simulink model "ss1_plant"  (R2019a)
settings: Solver=ode14x  StartTime=0  StopTime=0.456  FixedStep=1e-5  RelTol=1e-3  EnableMultiTasking=on
model workspace (MAT data in the model file):
  Ankle_L_D = 1.86999822456
  Ankle_L_S = 0.0237763920936
  Ankle_R_D = 0.0588397140494
  Ankle_R_S = 0.739584271752
  BeginTimePlantModel = 0.4399
  F_C = 0.06105
  F_H = 0.07
  F_I = 0.00125071180063
  F_L = 0.185
  F_M = 1.13129
  F_W = 0.1
  GRF_HD = 42097.5090581
  GRF_HS = 111995.804745
  GRF_VD = 23523.4518935
  GRF_VS = 88551.3661398
  HAT_I = 3.41998320224
  HAT_L = 0.51264
  HAT_M = 52.89756
  HAT_a = 0.2
  HAT_b = 0.11
  Hip_L_D = 0.00120944164738
  Hip_L_S = 1.91959156409
  Hip_R_D = 0.00174333284727
  Hip_R_S = 0.483982271561
  Knee_L_D = 0.900041230997
  Knee_L_S = 0.0187606009115
  Knee_R_D = 0.0722123401531
  Knee_R_S = 0.0187606009115
  M.stance_ankle = [382.653686523 421.133239746 457.361541748 493.224731445 525.049987793 550.694458008 572.993469238 598.336730957 620.458862305 635.94519043 652.86328125 671.32611084 ... (423 elements, 47x9)]
  M.swing_ankle = [-64.56690979 -57.5369148254 -49.8586082458 -42.14686203 -34.9792785645 -28.8147373199 -23.9411888123 -20.4650421143 -18.3295040131 -17.3495578766 -17.2596321106 -17.7645645142 ... (423 elements, 47x9)]
  M.stance_knee = [185.316421509 185.123703003 166.678710938 142.01902771 126.282310486 108.778045654 87.2157897949 52.3953895569 22.9555110931 -3.17964363098 -32.4531135559 -65.8174972534 ... (423 elements, 47x9)]
  M.swing_knee = [202.892730713 206.914764404 207.933639526 206.428604126 202.740692139 197.00177002 189.179733276 179.200378418 167.046905518 152.816116333 136.765853882 119.338562012 ... (423 elements, 47x9)]
  M.stance_hip = [670.444702148 608.623657227 559.095275879 508.654876709 434.052734375 368.594573975 310.278961182 279.085662842 245.949050903 213.394500732 182.434371948 163.658477783 ... (423 elements, 47x9)]
  M.swing_hip = [-409.603179932 -359.277313232 -304.840881348 -249.20954895 -195.251098633 -145.451843262 -101.693771362 -65.1620788574 -36.3202857971 -14.975810051 -0.45988124609 8.15607261658 ... (423 elements, 47x9)]
  M.stance_ankle_R = [241.344528198; 280.168792725; 315.234191895; 348.458496094; 375.407714844; 399.663421631; 420.77545166; 442.00982666; 462.368896484; 482.825683594; 502.481842041; 523.450317383; 543.702514648; 563.76739502; 584.623718262; 608.33001709; 633.130554199; 657.775634766; 683.749755859; 711.640380859; 738.552185059; 768.736328125; 798.939575195; 830.134277344; 862.95526123; 898.023254395; 934.645629883; 972.008911133; 1011.71954346; 1055.21350098; 1097.53088379; 1139.15075684; 1184.00402832; 1226.12475586; 1272.13769531; 1317.50842285; 1363.38061523; 1410.83459473; 1458.66088867; 1508.37402344; 1555.03942871; 1603.10827637; 1646.82128906; 1687.64489746; 1723.93286133; 1751.32250977; 1770.82592773]
  M.stance_ankle_L = [287.473602295; 320.288269043; 349.08013916; 375.086364746; 395.886169434; 413.086242676; 431.677429199; 447.653686523; 460.621368408; 476.93057251; 488.465698242; 501.313568115; 513.783081055; 527.231506348; 539.797363281; 552.587890625; 569.811767578; 585.799377441; 603.606445312; 624.266845703; 643.495849609; 666.619628906; 688.561279297; 712.704589844; 739.405578613; 766.059448242; 795.171264648; 824.763977051; 856.478515625; 892.682617188; 931.757080078; 975.575866699; 1018.39880371; 1068.90014648; 1121.41381836; 1177.15283203; 1233.20629883; 1294.38818359; 1356.3717041; 1418.45397949; 1482.10351562; 1546.63952637; 1606.78869629; 1662.24047852; 1713.70678711; 1755.8515625; 1788.09362793]
  M.stance_ankle_av = [261.846343994; 297.999664307; 330.276824951; 360.293121338; 384.509216309; 405.629089355; 425.620788574; 444.518188477; 461.592163086; 480.205688477; 496.252441406; 513.611755371; 530.404968262; 547.529174805; 564.700927734; 583.555786133; 604.988952637; 625.786193848; 648.130554199; 672.807739258; 696.304931641; 723.351074219; 749.882568359; 777.94329834; 808.044250488; 839.372680664; 872.657043457; 906.566711426; 942.723388672; 982.977416992; 1023.8536377; 1066.45080566; 1110.4017334; 1156.24707031; 1205.14941406; 1255.12817383; 1305.52526855; 1359.08056641; 1413.19909668; 1468.4095459; 1522.62353516; 1578.0111084; 1629.02905273; 1676.35400391; 1719.38793945; 1753.33544922; 1778.50048828]
  M.swing_ankle_R = [-85.889755249; -81.4323501587; -74.6266021729; -66.0338897705; -56.3612289429; -46.4022369385; -36.9383659363; -28.6265506744; -21.9128284454; -16.9965763092; -13.8461885452; -12.2523727417; -11.90001297; -12.4406614304; -13.5472927094; -14.9475679398; -16.441400528; -17.9046211243; -19.2776374817; -20.5434951782; -21.7070045471; -22.7848415375; -23.8007354736; -24.7754402161; -25.7178401947; -26.6206970215; -27.4531345367; -28.1520080566; -28.6213436127; -28.7432765961; -28.3963775635; -27.4741096497; -25.8983421326; -23.630197525; -20.6837310791; -17.1333255768; -13.1102085114; -8.78991889954; -4.37020587921; -0.0491741187871; 3.98967981339; 7.58726263046; 10.6098003387; 12.9361820221; 14.4380645752; 14.9655628204; 14.3451595306]
  M.swing_ankle_L = [-91.127494812; -88.5172576904; -83.079864502; -75.4265975952; -66.2622070312; -56.3544692993; -46.4767227173; -37.3417816162; -29.5312213898; -23.4348373413; -19.2079906464; -16.7372932434; -15.7042217255; -15.6731481552; -16.1855201721; -16.8559093475; -17.4320354462; -17.8048992157; -17.9840106964; -18.0637702942; -18.1733226776; -18.4301319122; -18.9239711761; -19.703086853; -20.7669734955; -22.0817985535; -23.5756607056; -25.1771774292; -26.8119258881; -28.3871974945; -29.7975158691; -30.9079360962; -31.557094574; -31.5594387054; -30.7291984558; -28.9196014404; -26.046585083; -22.1039409637; -17.1780376434; -11.4525842667; -5.19651222229; 1.25971031189; 7.55906391144; 13.3445072174; 18.2731304169; 22.0209007263; 23.2506732941]
  M.swing_ankle_av = [-88.2176361084; -84.5811920166; -78.3836135864; -70.2084197998; -60.7616653442; -50.8254547119; -41.1776351929; -32.4999885559; -25.2987804413; -19.8580245972; -16.2292098999; -14.2456712723; -13.5907716751; -13.877322197; -14.7198381424; -15.7957201004; -16.8816833496; -17.8603000641; -18.7026901245; -19.4413948059; -20.1364784241; -20.8494167328; -21.6332855225; -22.5210609436; -23.5174541473; -24.6034088135; -25.7298126221; -26.8298587799; -27.8171577454; -28.5850219727; -29.0191078186; -29.0002574921; -28.4133434296; -27.1543045044; -25.1483840942; -22.3716716766; -18.859708786; -14.7072620392; -10.0625753403; -5.11735677719; -0.093072257936; 4.77501726151; 9.25391769409; 13.1176586151; 16.142539978; 18.101266861; 18.3031654358]
  M.stance_knee_R = [304.803405762; 300.279541016; 286.749908447; 260.876068115; 238.10295105; 210.641204834; 181.547897339; 150.171356201; 117.616073608; 82.4058685303; 47.2514076233; 9.42407417297; -24.2061710358; -57.419593811; -89.7506561279; -121.374229431; -150.608276367; -177.107696533; -205.262542725; -233.704879761; -258.570648193; -287.401275635; -315.001159668; -341.735992432; -368.986816406; -397.352233887; -429.581481934; -461.832946777; -494.10635376; -527.185058594; -559.887207031; -588.972290039; -619.081665039; -645.119018555; -673.582641602; -697.401916504; -718.140319824; -735.778747559; -747.575012207; -758.092407227; -758.573730469; -756.998291016; -746.309448242; -733.501403809; -711.673217773; -684.145324707; -652.518432617]
  M.stance_knee_L = [243.44644165; 255.942733765; 248.447509766; 236.900390625; 224.860092163; 212.20489502; 192.68132019; 170.520477295; 148.683563232; 121.948730469; 95.7874603271; 68.55103302; 42.090297699; 13.6919345856; -12.3652801514; -38.7850036621; -64.9619522095; -88.0590744019; -112.283294678; -133.897094727; -155.896942139; -177.537506104; -199.712860107; -222.443725586; -246.961090088; -269.91027832; -297.39855957; -322.404815674; -347.004272461; -374.282318115; -397.260803223; -423.561889648; -443.694885254; -465.390808105; -484.542419434; -506.723937988; -523.60723877; -539.251403809; -553.182617188; -561.621337891; -567.393188477; -571.484802246; -571.686096191; -565.345947266; -556.19708252; -540.071105957; -519.244873047]
  M.stance_knee_av = [277.533630371; 280.574310303; 269.726623535; 250.220214844; 232.217224121; 211.336181641; 186.49609375; 159.215408325; 131.423858643; 99.98046875; 68.8229904175; 35.7027206421; 5.25892496109; -25.8144702911; -55.3571586609; -84.6679153442; -112.543243408; -137.530532837; -163.938446045; -189.345840454; -212.937911987; -238.572921753; -263.761932373; -288.717193604; -314.753173828; -340.711364746; -370.833557129; -399.864898682; -428.727661133; -459.228302002; -487.608825684; -515.456542969; -541.131958008; -565.239746094; -589.564758301; -612.656066895; -631.681152344; -648.433227539; -661.178405762; -670.771911621; -673.604614258; -674.547729492; -668.699035645; -658.765625; -642.572753906; -620.112365723; -593.285766602]
  M.swing_knee_R = [199.516082764; 210.401519775; 215.828033447; 216.27961731; 212.701660156; 206.257568359; 198.006378174; 188.676239014; 178.593338013; 167.751281738; 155.966705322; 143.082733154; 129.140670776; 114.425209045; 99.4022216797; 84.6166915894; 70.5888824463; 57.7218399048; 46.2420120239; 36.183429718; 27.4012203217; 19.5964603424; 12.3447122574; 5.1349864006; -2.6006064415; -11.4854259491; -22.1804237366; -35.3444290161; -51.6237678528; -71.6230010986; -95.8606109619; -124.642044067; -157.887771606; -194.970367432; -234.706756592; -275.472839355; -315.379730225; -352.45715332; -384.76776123; -410.475341797; -427.916656494; -435.71270752; -432.9347229; -419.276306152; -395.139343262; -361.678741455; -320.789794922]
  M.swing_knee_L = [164.096496582; 181.32963562; 193.40145874; 200.345535278; 202.785949707; 201.703689575; 198.146636963; 192.944168091; 186.504760742; 178.839569092; 169.754180908; 159.021072388; 146.566345215; 132.544692993; 117.362823486; 101.647209167; 86.1308898926; 71.517906189; 58.3772506714; 47.1123123169; 37.946975708; 30.9007816315; 25.7909584045; 22.2543544769; 19.7833538055; 17.7391624451; 15.3230056763; 11.6997699738; 6.09846830368; -2.1977686882; -13.9393539429; -29.9818992615; -51.2079772949; -78.3828964233; -111.999908447; -152.125411987; -198.241424561; -249.101135254; -302.666015625; -356.14050293; -406.130554199; -448.915588379; -480.807739258; -498.666107178; -500.297241211; -484.827392578; -454.950439453]
  M.swing_knee_av = [367.548095703; 394.961334229; 411.721313477; 418.395629883; 416.589355469; 408.467224121; 396.137420654; 381.146179199; 364.219024658; 345.358825684; 324.188934326; 300.332885742; 273.770843506; 244.956619263; 214.769424438; 184.371643066; 154.992874146; 127.706855774; 103.270904541; 82.0814208984; 64.1764450073; 49.2412033081; 36.6416435242; 25.4871902466; 14.6956396103; 3.0065600872; -5.51223230362; -14.4358959198; -25.9694404602; -40.7673416138; -59.4511642456; -82.5708694458; -110.474525452; -143.1537323; -180.170394897; -220.651763916; -263.318267822; -306.521148682; -348.278106689; -386.326507568; -418.233947754; -441.580657959; -454.211608887; -454.560668945; -441.876159668; -416.411499023; -380.416778564]
  M.stance_hip_R = [677.309082031; 662.534851074; 638.490905762; 616.795959473; 568.749938965; 517.141235352; 455.908843994; 395.977142334; 341.056732178; 296.010314941; 256.942687988; 232.045257568; 207.015548706; 187.887771606; 172.106338501; 157.565826416; 140.384109497; 121.182800293; 105.588790894; 91.3845062256; 72.1999969482; 60.2186164856; 45.7028198242; 30.413274765; 15.0268573761; 0.406857311726; -7.57483196259; -15.6972227097; -25.5365505219; -37.0106239319; -47.2925415039; -63.028678894; -78.3000335693; -97.126083374; -112.66633606; -133.688415527; -158.219207764; -186.10067749; -222.072463989; -257.30267334; -303.991699219; -349.784912109; -402.389801025; -448.147857666; -499.237121582; -543.315307617; -578.758666992]
  M.stance_hip_L = [543.206542969; 533.482299805; 548.817321777; 551.911437988; 531.989379883; 493.179870605; 449.218536377; 400.603149414; 345.233306885; 294.070343018; 246.907104492; 206.114685059; 169.324005127; 144.570343018; 122.85004425; 107.517539978; 94.4359436035; 78.0879211426; 64.8094940186; 47.6538200378; 33.5419006348; 17.3963489532; 5.34900474548; -6.64071655273; -16.2073192596; -27.9363861084; -31.1544418335; -38.8874778748; -46.7718048096; -50.9772720337; -62.9813499451; -70.4582366943; -86.7793121338; -104.007881165; -125.457344055; -142.477386475; -168.722595215; -199.240997314; -232.18812561; -274.7059021; -320.62008667; -367.697479248; -414.968200684; -465.465026855; -512.790344238; -558.792602539; -597.835327148]
  M.stance_hip_av = [617.707946777; 605.178161621; 598.635986328; 587.958374023; 552.411865234; 506.491699219; 452.935394287; 398.03314209; 342.912994385; 295.148101807; 252.482421875; 220.520568848; 190.263763428; 168.635574341; 150.214660645; 135.322143555; 119.96269989; 102.029510498; 87.4646606445; 71.9486465454; 55.0186271667; 41.1864967346; 27.767791748; 13.9448347092; 1.1450009346; -12.1901378632; -18.0546607971; -26.0040035248; -34.9744415283; -43.2180213928; -54.2653427124; -66.3307037354; -82.0686035156; -100.184661865; -118.351226807; -137.59463501; -162.887359619; -191.940826416; -226.568313599; -265.037445068; -311.382110596; -357.746063232; -407.980194092; -455.844390869; -505.260803223; -550.194091797; -587.237182617]
  M.swing_hip_R = [-538.103820801; -497.101409912; -442.370605469; -376.893707275; -304.863922119; -231.227020264; -160.946350098; -98.2951431274; -46.3001785278; -6.44236755371; 21.340795517; 38.314250946; 46.3760261536; 47.5502052307; 43.6576118469; 36.0970802307; 25.7352046967; 12.9887065887; -1.99190557003; -19.1645908356; -38.4166030884; -59.3577880859; -81.1436386108; -102.423095703; -121.337936401; -135.433135986; -141.69631958; -136.773361206; -117.19405365; -79.869178772; -22.6713924408; 54.7419433594; 150.165710449; 258.460906982; 372.17489624; 482.859954834; 582.569580078; 665.075012207; 726.33203125; 764.304260254; 778.477111816; 769.368469238; 738.280151367; 687.311401367; 619.35723877; 538.24987793; 448.937438965]
  M.swing_hip_L = [-461.667541504; -443.129730225; -412.952697754; -372.32824707; -323.551696777; -269.754852295; -214.532669067; -161.444091797; -113.441833496; -72.5716552734; -39.8347740173; -15.1222686768; 2.44718074799; 14.1845970154; 21.4651794434; 25.459356308; 27.0601558685; 26.8279724121; 24.9684696198; 21.2653636932; 15.2047595978; 6.27575731277; -5.8063416481; -20.9604568481; -38.6427841187; -57.7537269592; -76.4598388672; -92.4824371338; -103.319824219; -106.302307129; -98.579864502; -77.1716766357; -39.4084091187; 16.4871692657; 90.8427581787; 182.152694702; 286.93371582; 399.804718018; 513.893920898; 621.449401855; 714.596923828; 786.088867188; 829.926391602; 842.146728516; 821.168579102; 768.122131348; 691.412231445]
  M.swing_hip_av = [-504.132110596; -473.113983154; -429.29598999; -374.864593506; -313.169586182; -248.350509644; -184.762496948; -126.361343384; -76.1409072876; -35.8331642151; -5.84834623337; 14.5646886826; 26.8520946503; 32.7210464478; 33.7943077087; 31.3692054749; 26.3240718842; 19.1394901276; 9.99048233032; -1.19572210312; -14.5848884583; -30.1873207092; -47.6603965759; -66.2174758911; -84.5845413208; -100.908950806; -112.702316284; -117.088516235; -111.027740479; -91.6172332764; -56.4084892273; -3.88633561134; 65.9105529785; 150.917037964; 247.138397217; 349.212280273; 451.17590332; 547.177124023; 631.915161133; 700.813171387; 750.08581543; 776.799743652; 779.01184082; 756.12713623; 709.051147461; 640.415344238; 556.704040527]
  S_I = 0.0556212184297
  S_L = 0.41
  S_M = 3.62793
  S_R1 = 0.035
  S_R2 = 0.0716197243914
  T_I = 0.63371745
  T_L = 0.6
  T_M = 7.802
  T_R1 = 0.0716197243914
  T_R2 = 0.105042262441
  bodymass = 78.02
  p_stance_ankle = 3.52408223904
  p_stance_hip = 23.8147315857
  p_stance_knee = -14.6270017634
  p_swing_ankle = -34.807471817
  p_swing_hip = -19.0751814577
  p_swing_knee = -0.719736499265
  polyfit_stance_ankle = [7.25005766341 -2.94260084728 3.61751641686 -0.1600680665]
  polyfit_swing_ankle = [-11368.0037517 20285.4827832 -14825.218273 5697.61347658 -1221.0674564 140.988649334 -7.60353693637 0.110238664523]
  polyfit_swing_hip = [-6497.04836191 6353.1189755 -1512.41069047 -218.046365216 114.745718447 -9.14187395017 -0.14056630138]
  polyfit_swing_knee = [20801.7792641 -51031.8985583 53804.8965773 -29864.6420618 9069.83319333 -1458.09150169 107.955966741 -2.65469998779 0.0787369748099]
  stance_hip_D = -0.2
  stance_hip_I = 0
  stance_hip_P = -2
  stance_knee_D = 0.1
  stance_knee_I = 0
  stance_knee_P = 1
  u_stance_ankle = [2.09207920849e-06 2.83402277191e-05 -1.09458664945e-06 -2.15225634711e-07 1.00199670569e-07 -0.0321391439721]
  u_swing_ankle = [-0.000249118459232 -0.000670477458577 -0.000829633071132 -0.000874405796854 -0.000839016598733 -0.000796307977786]
  u_swing_hip = [-0.00160905629459 -0.00453587585235 -0.00786706006827 -0.000770525358696 -0.0150520831351 -0.0149081405775]
  u_swing_knee = [6.43563712018e-07 -4.04341590665e-07 7.15097641992e-07 -6.45757706781e-07 -0.0441867306802 -2.32579449741e-08]
  w_stance_ankle = 15.4408631407
  w_stance_hip = -43.933457531
  w_stance_knee = -25.2069201526
  w_swing_ankle = -15.2
  w_swing_hip = 136.9
  w_swing_knee = -386.2
undefined symbols (not defined in the file or in its folder): X, Y, Z
libraries: nesl_utility x81, sm_lib x49, fl_lib x24, fl_ps_legacy_lib x16
(part 1 of 7)
settings Model: OrderedModelArguments=off  Creator=6438sunj  LastModifiedBy=jess-local
settings DataIOCC: LimitDataPoints=on  SaveFormat=Array  SignalLoggingSaveFormat=ModelDataLogs  ReturnWorkspaceOutputs=off  SignalLoggingName=SPE_DataLog  OutputOption=SpecifiedOutputTimes  OutputTimes=spe_config.time
settings OptimizationCC: ExpressionDepthLimit=2147483647  LifeSpan=inf
settings DebuggingCC: UnderspecifiedInitializationDetection=Classic  MergeDetectMultiDrivingBlocksExec=none  SolverPrmCheckMsg=warning  StateNameClashWarn=warning  SFUnexpectedBacktrackingDiag=warning  SFNoUnconditionalDefaultTransitionDiag=warning  SFExecutionAtInitializationDiag=none  ArithmeticOperatorsInVariantConditions=warning
settings HardwareCC: ProdBitPerPointer=32  ProdBitPerSizeT=32  ProdBitPerPtrDiffT=32  ProdLargestAtomicFloat=None  ProdIntDivRoundTo=Undefined  ProdEndianess=Unspecified  ProdWordSize=32  ProdHWDeviceType=32-bit Generic
settings ModelReferenceCC: PropagateSignalLabelsOutOfModel=off
settings SFSimCC: SimUseLocalCustomCode=off
settings RTWCC: RTWUseLocalCustomCode=off
settings CodeAppCC: StateflowObjectComments=on
settings GRTTargetCC: TargetLangStandard=C89/C90 (ANSI)  GeneratePreprocessorConditionals=Disable all
settings ConfigComp: CovMetricSettings=dw  CovHtmlReporting=on  CovSaveCumulativeToWorkspaceVar=on  CovSaveSingleToWorkspaceVar=on  CovExternalEMLEnable=off
settings SimscapeCC: SimscapeNormalizeSystem=off
settings ConfigurationSet: Description=SimMechanics 2G
settings DiagnosticsConfigSet: SimMechanicsUnconnectedFramePorts=none
settings ExplorerConfigSet: InternalSimMechanicsExplorerSettings="<ExplorerConfiguration><canonicalview>default</canonicalview><TilePanel><TileInfo><Tiles Columns=\"1\" Count=\"1\" Rows=\"1\"><Column Left=\"2\" Weight=\"1\"/><Column Left=\"715\"/><Row Top=\"2\" Weight=\"1\"/><Row Top=\"555\"/><Tile Height=\"1\" Width=\"1\" X=\"0\" Y=\"0\"/></Tiles></TileInfo><SceneInfo><SceneViewer><BGColor><R>0.60000002384185791</R><G>0.60000002384185791</G><B>0.60000002384185791</B></BGColor><Camera><Position><X>2.3238188926266905</X><Y>0.29801581507321606</Y><Z>0.5830879823253462</Z></Position><Center><X>0</X><Y>0.29801581507321606</Y><Z>0.5830879823253462</Z></Center><Up><X>-0</X><Y>0</Y><Z>1</Z></Up><Left>-0.37797235250473021</Left><Right>0.37797235250473021</Right><Bottom>-0.82692947387695315</Bottom><Top>0.82692947387695315</Top></Camera></SceneViewer></SceneInfo></TilePanel></ExplorerConfiguration>"

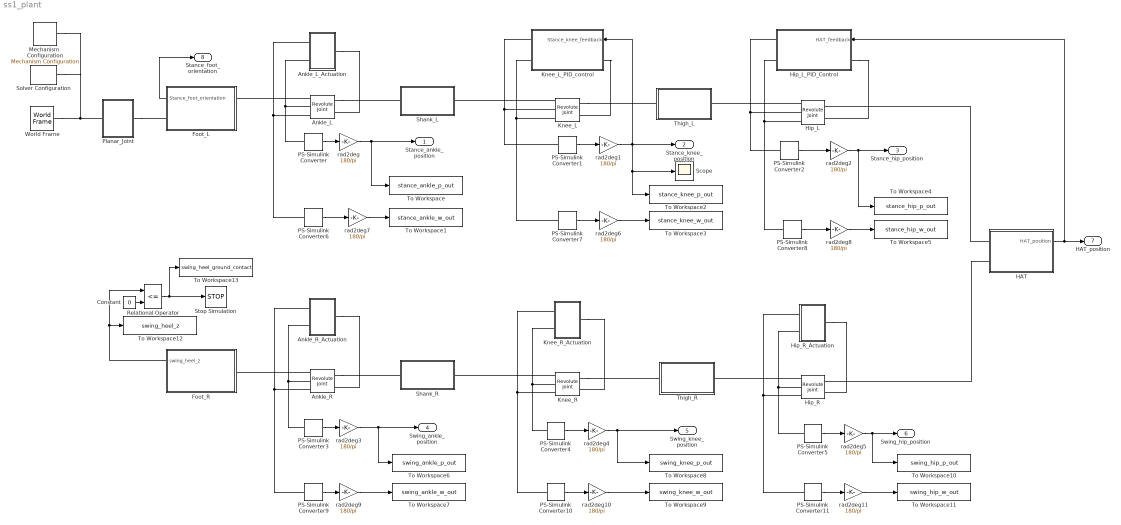
== system ss1_plant ==
  Ankle_L : sm_lib/Joints/Revolute Joint  SenseConstraintForce=off  SenseConstraintForceX=off  SenseConstraintForceY=off  SenseConstraintForceZ=off  SenseConstraintTorque=off  SenseConstraintTorqueX=off  SenseConstraintTorqueY=off  SenseConstraintTorqueZ=off  SenseTotalForce=off  SenseTotalForceX=off  SenseTotalForceY=off  SenseTotalForceZ=off  SenseTotalTorque=off  SenseTotalTorqueX=off  SenseTotalTorqueY=off  SenseTotalTorqueZ=off  CompositeWrenchDir=FollowerOnBase  CompositeWrenchFrame=BaseFrame  EquilibriumPosition=0  EquilibriumPositionUnits=deg  SpringStiffness=Ankle_L_S  SpringStiffnessUnits=N*m/deg  DampingCoefficient=Ankle_L_D  DampingCoefficientUnits=N*m/(deg/s)  TorqueActuationMode=InputTorque  MotionActuationMode=ComputedMotion  SensePosition=on  SenseVelocity=on  SenseAcceleration=off  SenseTorqueForce=off  SenseLowerLimitTorqueForce=off  SenseUpperLimitTorqueForce=off  LowerLimitSpecify=off  LowerLimitBound=-90  LowerLimitBoundUnits=deg  LowerLimitStiffness=1e4  LowerLimitStiffnessUnits=N*m/deg  LowerLimitDamping=10  LowerLimitDampingUnits=N*m/(deg/s)  LowerLimitTransitionRegionWidth=0.1  LowerLimitTransitionRegionWidthUnits=deg  UpperLimitSpecify=off  UpperLimitBound=90  UpperLimitBoundUnits=deg  UpperLimitStiffness=1e4  UpperLimitStiffnessUnits=N*m/deg  UpperLimitDamping=10  UpperLimitDampingUnits=N*m/(deg/s)  UpperLimitTransitionRegionWidth=0.1  UpperLimitTransitionRegionWidthUnits=deg  PositionTargetSpecify=on  PositionTargetPriority=High  PositionTargetValue=p_stance_ankle  PositionTargetValueUnits=deg  VelocityTargetSpecify=on  VelocityTargetPriority=High  VelocityTargetValue=w_stance_ankle  VelocityTargetValueUnits=deg/s
  Ankle_L_Actuation : Subsystem
  Ankle_R : sm_lib/Joints/Revolute Joint  SenseConstraintForce=off  SenseConstraintForceX=off  SenseConstraintForceY=off  SenseConstraintForceZ=off  SenseConstraintTorque=off  SenseConstraintTorqueX=off  SenseConstraintTorqueY=off  SenseConstraintTorqueZ=off  SenseTotalForce=off  SenseTotalForceX=off  SenseTotalForceY=off  SenseTotalForceZ=off  SenseTotalTorque=off  SenseTotalTorqueX=off  SenseTotalTorqueY=off  SenseTotalTorqueZ=off  CompositeWrenchDir=FollowerOnBase  CompositeWrenchFrame=BaseFrame  EquilibriumPosition=0  EquilibriumPositionUnits=deg  SpringStiffness=Ankle_R_S  SpringStiffnessUnits=N*m/deg  DampingCoefficient=Ankle_R_D  DampingCoefficientUnits=N*m/(deg/s)  TorqueActuationMode=InputTorque  MotionActuationMode=ComputedMotion  SensePosition=on  SenseVelocity=on  SenseAcceleration=off  SenseTorqueForce=off  SenseLowerLimitTorqueForce=off  SenseUpperLimitTorqueForce=off  LowerLimitSpecify=off  LowerLimitBound=-90  LowerLimitBoundUnits=deg  LowerLimitStiffness=1e4  LowerLimitStiffnessUnits=N*m/deg  LowerLimitDamping=10  LowerLimitDampingUnits=N*m/(deg/s)  LowerLimitTransitionRegionWidth=0.1  LowerLimitTransitionRegionWidthUnits=deg  UpperLimitSpecify=off  UpperLimitBound=90  UpperLimitBoundUnits=deg  UpperLimitStiffness=1e4  UpperLimitStiffnessUnits=N*m/deg  UpperLimitDamping=10  UpperLimitDampingUnits=N*m/(deg/s)  UpperLimitTransitionRegionWidth=0.1  UpperLimitTransitionRegionWidthUnits=deg  PositionTargetSpecify=on  PositionTargetPriority=High  PositionTargetValue=p_swing_ankle  PositionTargetValueUnits=deg  VelocityTargetSpecify=on  VelocityTargetPriority=High  VelocityTargetValue=w_swing_ankle  VelocityTargetValueUnits=deg/s
  Ankle_R_Actuation : Subsystem
  Constant : Constant  Value=0
  Foot_L : Subsystem  mask{F_L=F_L, F_H=F_H, F_C=F_C, F_W=F_W, F_M=F_M, F_I=F_I}
      mask prompts: F_L "Foot Length (m)"; F_H "Foot Height (m)"; F_C "Heel to Mid Foot (m)"; F_W "Foot Width (m)"; F_M "Foot Mass (kg)"; F_I "Foot Moment of Inertia (kg*m^2)"
      mask init:
      | % Defines the cross section of the thigh
      | 
      | F_cross_section = [(F_L-F_C),0;0, F_H; -F_C,0 ];
  Foot_R : Subsystem  mask{F_L=F_L, F_H=F_H, F_C=F_C, F_W=F_W, F_M=F_M, F_I=F_I}
      mask prompts: F_L "Foot Length (m)"; F_H "Foot Height (m)"; F_C "Heel to Mid Foot (m)"; F_W "Foot Width (m)"; F_M "Foot Mass (kg)"; F_I "Foot Moment of Inertia (kg*m^2)"
      mask init:
      | % Defines the cross section of the thigh
      | 
      | F_cross_section = [(F_L-F_C),0;0, F_H; -F_C,0; ];
  HAT : Subsystem  mask{HAT_a=HAT_a, HAT_b=HAT_b, HAT_L=HAT_L, HAT_M=HAT_M, HAT_I=HAT_I}
      mask prompts: HAT_a "Long Axis Length (m)"; HAT_b "Short Axis Length (m)"; HAT_L "HAT Height (m)"; HAT_M "Mass (kg)"; HAT_I "Moment of Inertia (kg*m^2)"
      mask init:
      | % Defines the cross-section of the HAT
      | theta = ([0:.01:360]*(pi/180))';
      | HAT_cross_section = [HAT_a*cos(theta), HAT_b*sin(theta)];
  Hip_L : sm_lib/Joints/Revolute Joint  SenseConstraintForce=off  SenseConstraintForceX=off  SenseConstraintForceY=off  SenseConstraintForceZ=off  SenseConstraintTorque=off  SenseConstraintTorqueX=off  SenseConstraintTorqueY=off  SenseConstraintTorqueZ=off  SenseTotalForce=off  SenseTotalForceX=off  SenseTotalForceY=off  SenseTotalForceZ=off  SenseTotalTorque=off  SenseTotalTorqueX=off  SenseTotalTorqueY=off  SenseTotalTorqueZ=off  CompositeWrenchDir=FollowerOnBase  CompositeWrenchFrame=BaseFrame  EquilibriumPosition=0  EquilibriumPositionUnits=deg  SpringStiffness=Hip_L_S  SpringStiffnessUnits=N*m/deg  DampingCoefficient=Hip_L_D  DampingCoefficientUnits=N*m/(deg/s)  TorqueActuationMode=InputTorque  MotionActuationMode=ComputedMotion  SensePosition=on  SenseVelocity=on  SenseAcceleration=off  SenseTorqueForce=off  SenseLowerLimitTorqueForce=off  SenseUpperLimitTorqueForce=off  LowerLimitSpecify=off  LowerLimitBound=-90  LowerLimitBoundUnits=deg  LowerLimitStiffness=1e4  LowerLimitStiffnessUnits=N*m/deg  LowerLimitDamping=10  LowerLimitDampingUnits=N*m/(deg/s)  LowerLimitTransitionRegionWidth=0.1  LowerLimitTransitionRegionWidthUnits=deg  UpperLimitSpecify=off  UpperLimitBound=90  UpperLimitBoundUnits=deg  UpperLimitStiffness=1e4  UpperLimitStiffnessUnits=N*m/deg  UpperLimitDamping=10  UpperLimitDampingUnits=N*m/(deg/s)  UpperLimitTransitionRegionWidth=0.1  UpperLimitTransitionRegionWidthUnits=deg  PositionTargetSpecify=on  PositionTargetPriority=High  PositionTargetValue=p_stance_hip  PositionTargetValueUnits=deg  VelocityTargetSpecify=on  VelocityTargetPriority=High  VelocityTargetValue=w_stance_hip  VelocityTargetValueUnits=deg/s
  Hip_L_PID_Control : Subsystem
  Hip_R : sm_lib/Joints/Revolute Joint  SenseConstraintForce=off  SenseConstraintForceX=off  SenseConstraintForceY=off  SenseConstraintForceZ=off  SenseConstraintTorque=off  SenseConstraintTorqueX=off  SenseConstraintTorqueY=off  SenseConstraintTorqueZ=off  SenseTotalForce=off  SenseTotalForceX=off  SenseTotalForceY=off  SenseTotalForceZ=off  SenseTotalTorque=off  SenseTotalTorqueX=off  SenseTotalTorqueY=off  SenseTotalTorqueZ=off  CompositeWrenchDir=FollowerOnBase  CompositeWrenchFrame=BaseFrame  EquilibriumPosition=0  EquilibriumPositionUnits=deg  SpringStiffness=Hip_R_S  SpringStiffnessUnits=N*m/deg  DampingCoefficient=Hip_R_D  DampingCoefficientUnits=N*m/(deg/s)  TorqueActuationMode=InputTorque  MotionActuationMode=ComputedMotion  SensePosition=on  SenseVelocity=on  SenseAcceleration=off  SenseTorqueForce=off  SenseLowerLimitTorqueForce=off  SenseUpperLimitTorqueForce=off  LowerLimitSpecify=off  LowerLimitBound=-90  LowerLimitBoundUnits=deg  LowerLimitStiffness=1e4  LowerLimitStiffnessUnits=N*m/deg  LowerLimitDamping=10  LowerLimitDampingUnits=N*m/(deg/s)  LowerLimitTransitionRegionWidth=0.1  LowerLimitTransitionRegionWidthUnits=deg  UpperLimitSpecify=off  UpperLimitBound=90  UpperLimitBoundUnits=deg  UpperLimitStiffness=1e4  UpperLimitStiffnessUnits=N*m/deg  UpperLimitDamping=10  UpperLimitDampingUnits=N*m/(deg/s)  UpperLimitTransitionRegionWidth=0.1  UpperLimitTransitionRegionWidthUnits=deg  PositionTargetSpecify=on  PositionTargetPriority=High  PositionTargetValue=p_swing_hip  PositionTargetValueUnits=deg  VelocityTargetSpecify=on  VelocityTargetPriority=High  VelocityTargetValue=w_swing_hip  VelocityTargetValueUnits=deg/s
  Hip_R_Actuation : Subsystem
  Knee_L : sm_lib/Joints/Revolute Joint  SenseConstraintForce=off  SenseConstraintForceX=off  SenseConstraintForceY=off  SenseConstraintForceZ=off  SenseConstraintTorque=off  SenseConstraintTorqueX=off  SenseConstraintTorqueY=off  SenseConstraintTorqueZ=off  SenseTotalForce=off  SenseTotalForceX=off  SenseTotalForceY=off  SenseTotalForceZ=off  SenseTotalTorque=off  SenseTotalTorqueX=off  SenseTotalTorqueY=off  SenseTotalTorqueZ=off  CompositeWrenchDir=FollowerOnBase  CompositeWrenchFrame=BaseFrame  EquilibriumPosition=0  EquilibriumPositionUnits=deg  SpringStiffness=Knee_L_S  SpringStiffnessUnits=N*m/deg  DampingCoefficient=Knee_L_D  DampingCoefficientUnits=N*m/(deg/s)  TorqueActuationMode=InputTorque  MotionActuationMode=ComputedMotion  SensePosition=on  SenseVelocity=on  SenseAcceleration=off  SenseTorqueForce=off  SenseLowerLimitTorqueForce=off  SenseUpperLimitTorqueForce=off  LowerLimitSpecify=off  LowerLimitBound=-90  LowerLimitBoundUnits=deg  LowerLimitStiffness=1e4  LowerLimitStiffnessUnits=N*m/deg  LowerLimitDamping=10  LowerLimitDampingUnits=N*m/(deg/s)  LowerLimitTransitionRegionWidth=0.1  LowerLimitTransitionRegionWidthUnits=deg  UpperLimitSpecify=off  UpperLimitBound=90  UpperLimitBoundUnits=deg  UpperLimitStiffness=1e4  UpperLimitStiffnessUnits=N*m/deg  UpperLimitDamping=10  UpperLimitDampingUnits=N*m/(deg/s)  UpperLimitTransitionRegionWidth=0.1  UpperLimitTransitionRegionWidthUnits=deg  PositionTargetSpecify=on  PositionTargetPriority=High  PositionTargetValue=p_stance_knee  PositionTargetValueUnits=deg  VelocityTargetSpecify=on  VelocityTargetPriority=High  VelocityTargetValue=w_stance_knee  VelocityTargetValueUnits=deg/s
  Knee_L_PID_control : Subsystem
  Knee_R : sm_lib/Joints/Revolute Joint  SenseConstraintForce=off  SenseConstraintForceX=off  SenseConstraintForceY=off  SenseConstraintForceZ=off  SenseConstraintTorque=off  SenseConstraintTorqueX=off  SenseConstraintTorqueY=off  SenseConstraintTorqueZ=off  SenseTotalForce=off  SenseTotalForceX=off  SenseTotalForceY=off  SenseTotalForceZ=off  SenseTotalTorque=off  SenseTotalTorqueX=off  SenseTotalTorqueY=off  SenseTotalTorqueZ=off  CompositeWrenchDir=FollowerOnBase  CompositeWrenchFrame=BaseFrame  EquilibriumPosition=0  EquilibriumPositionUnits=deg  SpringStiffness=Knee_R_S  SpringStiffnessUnits=N*m/deg  DampingCoefficient=Knee_R_D  DampingCoefficientUnits=N*m/(deg/s)  TorqueActuationMode=InputTorque  MotionActuationMode=ComputedMotion  SensePosition=on  SenseVelocity=on  SenseAcceleration=off  SenseTorqueForce=off  SenseLowerLimitTorqueForce=off  SenseUpperLimitTorqueForce=off  LowerLimitSpecify=off  LowerLimitBound=-90  LowerLimitBoundUnits=deg  LowerLimitStiffness=1e4  LowerLimitStiffnessUnits=N*m/deg  LowerLimitDamping=10  LowerLimitDampingUnits=N*m/(deg/s)  LowerLimitTransitionRegionWidth=0.1  LowerLimitTransitionRegionWidthUnits=deg  UpperLimitSpecify=off  UpperLimitBound=90  UpperLimitBoundUnits=deg  UpperLimitStiffness=1e4  UpperLimitStiffnessUnits=N*m/deg  UpperLimitDamping=10  UpperLimitDampingUnits=N*m/(deg/s)  UpperLimitTransitionRegionWidth=0.1  UpperLimitTransitionRegionWidthUnits=deg  PositionTargetSpecify=on  PositionTargetPriority=High  PositionTargetValue=p_swing_knee  PositionTargetValueUnits=deg  VelocityTargetSpecify=on  VelocityTargetPriority=High  VelocityTargetValue=w_swing_knee  VelocityTargetValueUnits=deg/s
  Knee_R_Actuation : Subsystem
  Mechanism  Configuration : sm_lib/Utilities/Mechanism Configuration  UniformGravity=Constant  GravityVector=[0 0 -9.81]  GravityUnits=m/s^2  LinearizationDelta=0.001
  PS-Simulink Converter{,1..11} (12 alike) : nesl_utility/PS-Simulink Converter  PhysicalDomain=network_engine_domain  SubClassName=ps_output  LeftPortType=input  RightPortType=output  PseudoPeriodic=off  Frequencies=[]  Unit=1  AffineConversion=off
  Planar_Joint : Subsystem
  Relational Operator : RelationalOperator  Operator=<=  OutDataTypeStr=boolean  RndMeth=Simplest
  Scope : Scope
  Shank_L : Subsystem  mask{S_R2=S_R2, S_R1=S_R1, S_L=S_L, S_M=S_M, S_I=S_I}
      mask prompts: S_R2 "Proximal End Radius (m)"; S_R1 "Distal End Radius (m)"; S_L "Shank Length (m)"; S_M "Shank Mass (kg)"; S_I "Shank Moment of Inertia (kg*m^2)"
      mask init:
      | % Defines the cross section of the thigh
      | 
      | S_cross_section = [0,0; S_R1, 0; S_R2, S_L; 0,S_L];
  Shank_R : Subsystem  mask{S_R2=S_R2, S_R1=S_R1, S_L=S_L, S_M=S_M, S_I=S_I}
      mask prompts: S_R2 "Proximal End Radius (m)"; S_R1 "Distal End Radius (m)"; S_L "Shank Length (m)"; S_M "Shank Mass (kg)"; S_I "Shank Moment of Inertia (kg*m^2)"
      mask init:
      | % Defines the cross section of the thigh
      | 
      | S_cross_section = [0,0; S_R1, 0; S_R2, S_L; 0,S_L];
  Solver Configuration : nesl_utility/Solver Configuration  PhysicalDomain=network_engine_domain  SubClassName=solver  LeftPortType=input  RightPortType=generic  Tones=[]  Harmonics=[]  SimulateNoise=off  Profile=off  UseLocalSampling=off  EnableSwitchedLinearOptims=on  FrequencyDomain=off  UseCCode=off  RelTol=0.001  AbsTol=1e-06  MinStep=1e-09  ToWorkspace=off  RevertToSquareIcSolve=off  NumHomotopyIterations=100  PhasorMode=off  PhasorModeNumHarmonics=1  DoDC=off  ResidualTolerance=1e-9  UseLocalSolver=off  LocalSolverChoice=NE_BACKWARD_EULER_ADVANCER  LocalSolverSampleTime=.001  DoFixedCost=off  MaxNonlinIter=3  MaxModeIter=2  LinearAlgebra=Sparse  EquationFormulation=NE_TIME_EF  DelaysMemoryBudget=1024  AutomaticFiltering=on  FilteringTimeConstant=0.001  PartitionStorageMethod=AS_NEEDED  PartitionMemoryBudget=1024  PartitionMethod=FAST
  Stop Simulation : Stop
  Thigh_L : Subsystem  mask{T_R2=T_R2, T_R1=T_R1, T_L=T_L, T_M=T_M, T_I=T_I}
      mask prompts: T_R2 "Proximal End Radius (m)"; T_R1 "Distal End Radius (m)"; T_L "Thigh Length (m)"; T_M "Thigh Mass (kg)"; T_I "Thigh Moment of Inertia (kg*m^2)"
      mask init:
      | % Defines the cross section of the thigh
      | 
      | T_cross_section = [0,0; T_R1, 0; T_R2, T_L; 0,T_L];
  Thigh_R : Subsystem  mask{T_R2=T_R2, T_R1=T_R1, T_L=T_L, T_M=T_M, T_I=T_I}
      mask prompts: T_R2 "Proximal End Radius (m)"; T_R1 "Distal End Radius (m)"; T_L "Thigh Length (m)"; T_M "Thigh Mass (kg)"; T_I "Thigh Moment of Inertia (kg*m^2)"
      mask init:
      | % Defines the cross section of the thigh
      | 
      | T_cross_section = [0,0; T_R1, 0; T_R2, T_L; 0,T_L];
  To Workspace : ToWorkspace  VariableName=stance_ankle_p_out  SampleTime=-1
  To Workspace1 : ToWorkspace  VariableName=stance_ankle_w_out  SampleTime=-1
  To Workspace10 : ToWorkspace  VariableName=swing_hip_p_out  SampleTime=-1
  To Workspace11 : ToWorkspace  VariableName=swing_hip_w_out  SampleTime=-1
  To Workspace12 : ToWorkspace  VariableName=swing_heel_z  SampleTime=-1
  To Workspace13 : ToWorkspace  VariableName=swing_heel_ground_contact  SampleTime=-1
  To Workspace2 : ToWorkspace  VariableName=stance_knee_p_out  SampleTime=-1
  To Workspace3 : ToWorkspace  VariableName=stance_knee_w_out  SampleTime=-1
  To Workspace4 : ToWorkspace  VariableName=stance_hip_p_out  SampleTime=-1
  To Workspace5 : ToWorkspace  VariableName=stance_hip_w_out  SampleTime=-1
  To Workspace6 : ToWorkspace  VariableName=swing_ankle_p_out  SampleTime=-1
  To Workspace7 : ToWorkspace  VariableName=swing_ankle_w_out  SampleTime=-1
  To Workspace8 : ToWorkspace  VariableName=swing_knee_p_out  SampleTime=-1
  To Workspace9 : ToWorkspace  VariableName=swing_knee_w_out  SampleTime=-1
  World Frame : sm_lib/Frames and Transforms/World Frame
  rad2deg{,1..11} (12 alike) : Gain  Gain=180/pi
  Stance_ankle_position : Outport
  Stance_knee_position : Outport  Port=2
  Stance_hip_position : Outport  Port=3
  Swing_ankle_position : Outport  Port=4
  Swing_knee_position : Outport  Port=5
  Swing_hip_position : Outport  Port=6
  HAT_position : Outport  Port=7
  Stance_foot_orientation : Outport  Port=8
  wires:
  PS-Simulink Converter/1 -> rad2deg/1
  PS-Simulink Converter1/1 -> rad2deg1/1
  PS-Simulink Converter2/1 -> rad2deg2/1
  PS-Simulink Converter3/1 -> rad2deg3/1
  PS-Simulink Converter4/1 -> rad2deg4/1
  PS-Simulink Converter5/1 -> rad2deg5/1
  rad2deg/1 -> To Workspace/1, Stance_ankle_position/1
  rad2deg1/1 -> Knee_L_PID_control/1(Stance_knee_feedback), Scope/1, To Workspace2/1, Stance_knee_position/1
  rad2deg2/1 -> To Workspace4/1, Stance_hip_position/1
  rad2deg3/1 -> To Workspace6/1, Swing_ankle_position/1
  rad2deg4/1 -> To Workspace8/1, Swing_knee_position/1
  rad2deg5/1 -> To Workspace10/1, Swing_hip_position/1
  HAT/1(HAT_position) -> HAT_position/1, Hip_L_PID_Control/1(HAT_feedback)
  Foot_L/1(Stance_foot_orientation) -> Stance_foot_orientation/1
  PS-Simulink Converter6/1 -> rad2deg7/1
  rad2deg7/1 -> To Workspace1/1
  PS-Simulink Converter7/1 -> rad2deg6/1
  rad2deg6/1 -> To Workspace3/1
  PS-Simulink Converter8/1 -> rad2deg8/1
  rad2deg8/1 -> To Workspace5/1
  PS-Simulink Converter9/1 -> rad2deg9/1
  rad2deg9/1 -> To Workspace7/1
  PS-Simulink Converter10/1 -> rad2deg10/1
  rad2deg10/1 -> To Workspace9/1
  PS-Simulink Converter11/1 -> rad2deg11/1
  rad2deg11/1 -> To Workspace11/1
  Constant/1 -> Relational Operator/2
  Relational Operator/1 -> Stop Simulation/1, To Workspace13/1
  Foot_R/1(swing_heel_z) -> To Workspace12/1, Relational Operator/1
  connections:
  World Frame/RConn1 -- Mechanism  Configuration/RConn1 -- Solver Configuration/RConn1 -- Planar_Joint/LConn1
  Planar_Joint/RConn1 -- Foot_L/RConn1
  Ankle_L/RConn1 -- Foot_L/LConn1
  Ankle_L/LConn1 -- Shank_L/RConn1
  Knee_L/RConn1 -- Shank_L/LConn1
  Knee_L/LConn1 -- Thigh_L/RConn1
  Hip_L/RConn1 -- Thigh_L/LConn1
  HAT/LConn1 -- Hip_L/LConn1
  Ankle_R/RConn1 -- Foot_R/LConn1
  Ankle_R/LConn1 -- Shank_R/RConn1
  Knee_R/RConn1 -- Shank_R/LConn1
  Knee_R/LConn1 -- Thigh_R/RConn1
  Hip_R/RConn1 -- Thigh_R/LConn1
  HAT/LConn2 -- Hip_R/LConn1
  Ankle_L_Actuation/LConn1 -- Ankle_L/LConn2
  Ankle_L/RConn3 -- PS-Simulink Converter6/LConn1 -- Ankle_L_Actuation/RConn1
  Ankle_R/RConn3 -- PS-Simulink Converter9/LConn1 -- Ankle_R_Actuation/RConn1
  Knee_L/RConn3 -- Knee_L_PID_control/RConn2 -- PS-Simulink Converter7/LConn1
  Knee_R/RConn3 -- PS-Simulink Converter10/LConn1 -- Knee_R_Actuation/RConn1
  Hip_L/RConn3 -- PS-Simulink Converter8/LConn1 -- Hip_L_PID_Control/RConn2
  Hip_R/RConn3 -- PS-Simulink Converter11/LConn1 -- Hip_R_Actuation/RConn1
  Ankle_L/RConn2 -- Ankle_L_Actuation/RConn2 -- PS-Simulink Converter/LConn1
  Knee_L/RConn2 -- PS-Simulink Converter1/LConn1 -- Knee_L_PID_control/RConn1
  Hip_L/RConn2 -- Hip_L_PID_Control/RConn1 -- PS-Simulink Converter2/LConn1
  Ankle_R/RConn2 -- PS-Simulink Converter3/LConn1 -- Ankle_R_Actuation/RConn2
  Knee_R/RConn2 -- Knee_R_Actuation/RConn2 -- PS-Simulink Converter4/LConn1
  Hip_R/RConn2 -- PS-Simulink Converter5/LConn1 -- Hip_R_Actuation/RConn2
  Knee_L_PID_control/LConn1 -- Knee_L/LConn2
  Hip_L_PID_Control/LConn1 -- Hip_L/LConn2
  Hip_R_Actuation/LConn1 -- Hip_R/LConn2
  Knee_R_Actuation/LConn1 -- Knee_R/LConn2
  Ankle_R_Actuation/LConn1 -- Ankle_R/LConn2

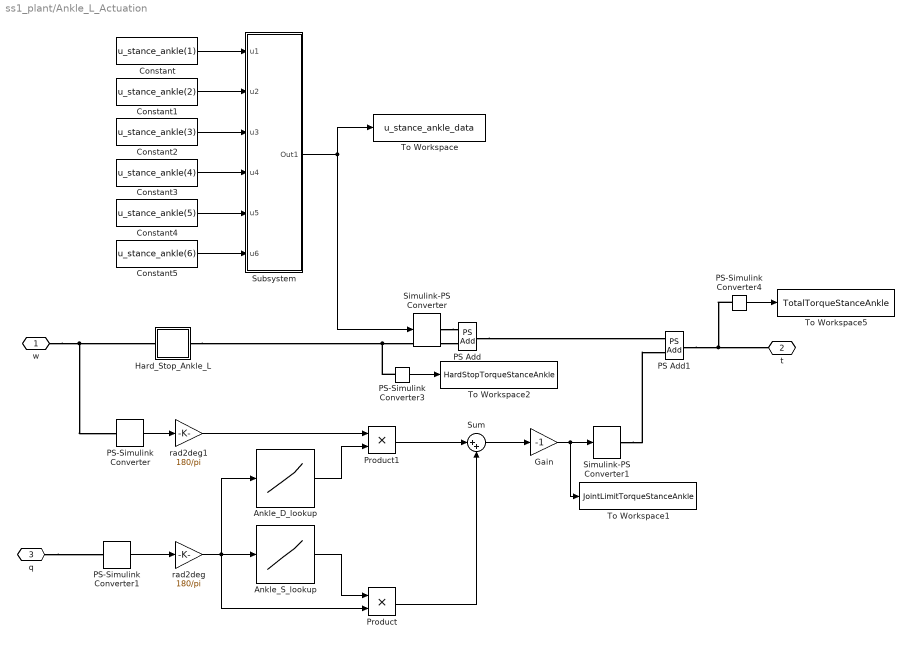
== system ss1_plant/Ankle_L_Actuation ==
  Ankle_D_lookup : Lookup_n-D  NumberOfTableDimensions=1  BreakpointsForDimension1=[-45:.01:20]  Table=[exp(linspace(log(1000),log(.01),1000)), zeros(1,4500),exp(linspace(log(.01),log(1000),1001))]  RndMeth=Simplest  InputSameDT=on
  Ankle_S_lookup : Lookup_n-D  NumberOfTableDimensions=1  BreakpointsForDimension1=[-45:.01:20]  Table=[exp(linspace(log(10000),log(.01),1000)), zeros(1,4500),exp(linspace(log(.01),log(10000),1001))]  RndMeth=Simplest  InputSameDT=on
  Constant : Constant  Value=u_stance_ankle(1)
  Constant1 : Constant  Value=u_stance_ankle(2)
  Constant2 : Constant  Value=u_stance_ankle(3)
  Constant3 : Constant  Value=u_stance_ankle(4)
  Constant4 : Constant  Value=u_stance_ankle(5)
  Constant5 : Constant  Value=u_stance_ankle(6)
  Gain : Gain  Gain=-1
  Hard_Stop_Ankle_L : Subsystem  mask{upper_bound=((20-p_stance_ankle)*pi)/180, lower_bound=((-45-p_stance_ankle)*pi)/180, contact_stiffness=1e8, contact_damping=5000, initial_angular_position=0}
      mask prompts: upper_bound "Upper Bound"; lower_bound "Lower Bound"; contact_stiffness "Contact Stiffness"; contact_damping "Contact Damping"; initial_angular_position "Initial Angular Position"
  PS Add : fl_ps_legacy_lib/Legacy Physical Signals/Functions/PS Add
      settings: SourceProductName=Simscape  SourceProductBaseCode=SS
  PS Add1 : fl_ps_legacy_lib/Legacy Physical Signals/Functions/PS Add
      settings: SourceProductName=Simscape  SourceProductBaseCode=SS
  PS-Simulink Converter{,1,3..4} (4 alike) : nesl_utility/PS-Simulink Converter  PhysicalDomain=network_engine_domain  SubClassName=ps_output  LeftPortType=input  RightPortType=output  PseudoPeriodic=off  Frequencies=[]  Unit=1  AffineConversion=off
  Product : Product  RndMeth=Zero
  Product1 : Product  RndMeth=Zero
  Simulink-PS Converter : nesl_utility/Simulink-PS Converter  PhysicalDomain=network_engine_domain  SubClassName=ps_input  LeftPortType=input  RightPortType=output  PseudoPeriodic=off  Frequencies=[]  NoiseDistribution=none  NoiseParameters=[]  Unit=1  AffineConversion=off  FilteringAndDerivatives=zero  SimscapeFilterOrder=1  InputFilterTimeConstant=.001  UdotUserProvided=[]
  Simulink-PS Converter1 : nesl_utility/Simulink-PS Converter  PhysicalDomain=network_engine_domain  SubClassName=ps_input  LeftPortType=input  RightPortType=output  PseudoPeriodic=off  Frequencies=[]  NoiseDistribution=none  NoiseParameters=[]  Unit=1  AffineConversion=off  FilteringAndDerivatives=zero  SimscapeFilterOrder=1  InputFilterTimeConstant=.001  UdotUserProvided=[]
  Subsystem : Subsystem
  Sum : Sum  Inputs=|++
  To Workspace : ToWorkspace  VariableName=u_stance_ankle_data  SampleTime=-1
  To Workspace1 : ToWorkspace  VariableName=JointLimitTorqueStanceAnkle  SampleTime=-1
  To Workspace2 : ToWorkspace  VariableName=HardStopTorqueStanceAnkle  SampleTime=-1
  To Workspace5 : ToWorkspace  VariableName=TotalTorqueStanceAnkle  SampleTime=-1
  rad2deg : Gain  Gain=180/pi
  "rad2deg1 " : Gain  Gain=180/pi
  w : PMIOPort  Side=Right
  t : PMIOPort  Port=2  Side=Left
  q : PMIOPort  Port=3  Side=Right
  wires:
  PS-Simulink Converter/1 -> "rad2deg1 "/1
  PS-Simulink Converter1/1 -> rad2deg/1
  rad2deg/1 -> Ankle_D_lookup/1, Product/2, Ankle_S_lookup/1
  Ankle_S_lookup/1 -> Product/1
  "rad2deg1 "/1 -> Product1/1
  Product1/1 -> Sum/1
  Product/1 -> Sum/2
  Sum/1 -> Gain/1
  Gain/1 -> To Workspace1/1, Simulink-PS Converter1/1
  Ankle_D_lookup/1 -> Product1/2
  Constant/1 -> Subsystem/1(u1)
  Constant1/1 -> Subsystem/2(u2)
  Constant2/1 -> Subsystem/3(u3)
  Constant3/1 -> Subsystem/4(u4)
  Constant4/1 -> Subsystem/5(u5)
  Subsystem/1(Out1) -> Simulink-PS Converter/1, To Workspace/1
  Constant5/1 -> Subsystem/6(u6)
  PS-Simulink Converter4/1 -> To Workspace5/1
  PS-Simulink Converter3/1 -> To Workspace2/1
  connections:
  w/RConn1 -- PS-Simulink Converter/LConn1 -- Hard_Stop_Ankle_L/LConn1
  Hard_Stop_Ankle_L/RConn1 -- PS-Simulink Converter3/LConn1 -- PS Add/LConn2
  q/RConn1 -- PS-Simulink Converter1/LConn1
  Simulink-PS Converter1/RConn1 -- PS Add1/LConn2
  PS Add/RConn1 -- PS Add1/LConn1
  PS Add1/RConn1 -- PS-Simulink Converter4/LConn1 -- t/RConn1
  Simulink-PS Converter/RConn1 -- PS Add/LConn1

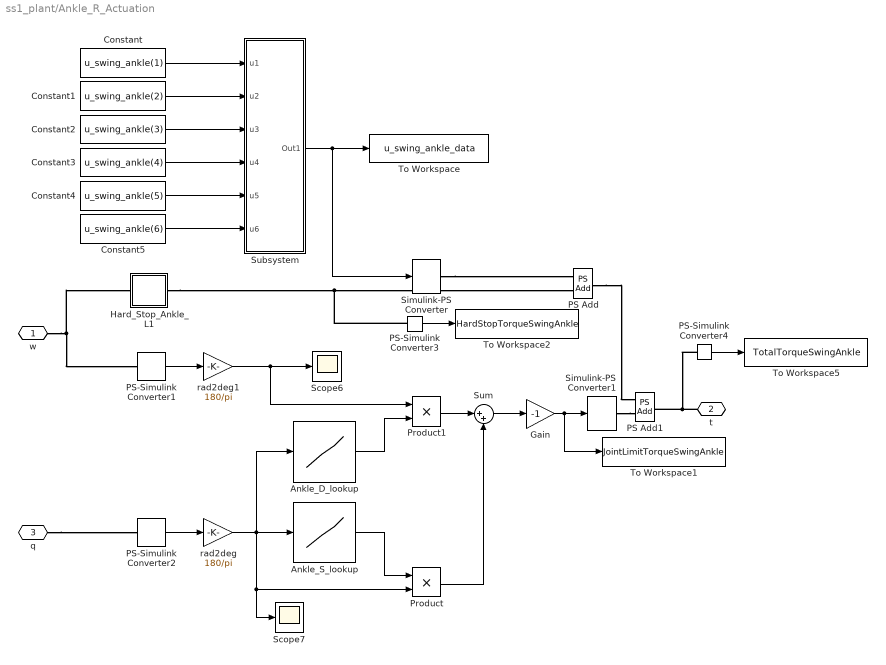
== system ss1_plant/Ankle_R_Actuation ==
  Ankle_D_lookup : Lookup_n-D  NumberOfTableDimensions=1  BreakpointsForDimension1=[-45:.01:20]  Table=[exp(linspace(log(1000),log(.01),1000)), zeros(1,4500),exp(linspace(log(.01),log(1000),1001))]  RndMeth=Simplest  InputSameDT=on
  Ankle_S_lookup : Lookup_n-D  NumberOfTableDimensions=1  BreakpointsForDimension1=[-45:.01:20]  Table=[exp(linspace(log(10000),log(.01),1000)), zeros(1,4500),exp(linspace(log(.01),log(10000),1001))]  RndMeth=Simplest  InputSameDT=on
  Constant : Constant  Value=u_swing_ankle(1)
  Constant1 : Constant  Value=u_swing_ankle(2)
  Constant2 : Constant  Value=u_swing_ankle(3)
  Constant3 : Constant  Value=u_swing_ankle(4)
  Constant4 : Constant  Value=u_swing_ankle(5)
  Constant5 : Constant  Value=u_swing_ankle(6)
  Gain : Gain  Gain=-1
  Hard_Stop_Ankle_L1 : Subsystem  mask{upper_bound=((20-p_swing_ankle)*pi)/180, lower_bound=((-45-p_swing_ankle)*pi)/180, contact_stiffness=1e8, contact_damping=5000, initial_angular_position=0}
      mask prompts: upper_bound "Upper Bound"; lower_bound "Lower Bound"; contact_stiffness "Contact Stiffness"; contact_damping "Contact Damping"; initial_angular_position "Initial Angular Position"
  PS Add : fl_ps_legacy_lib/Legacy Physical Signals/Functions/PS Add
      settings: SourceProductName=Simscape  SourceProductBaseCode=SS
  PS Add1 : fl_ps_legacy_lib/Legacy Physical Signals/Functions/PS Add
      settings: SourceProductName=Simscape  SourceProductBaseCode=SS
  PS-Simulink Converter{1..4} (4 alike) : nesl_utility/PS-Simulink Converter  PhysicalDomain=network_engine_domain  SubClassName=ps_output  LeftPortType=input  RightPortType=output  PseudoPeriodic=off  Frequencies=[]  Unit=1  AffineConversion=off
  Product : Product  RndMeth=Zero
  Product1 : Product  RndMeth=Zero
  Scope6 : Scope
  Scope7 : Scope
  Simulink-PS Converter : nesl_utility/Simulink-PS Converter  PhysicalDomain=network_engine_domain  SubClassName=ps_input  LeftPortType=input  RightPortType=output  PseudoPeriodic=off  Frequencies=[]  NoiseDistribution=none  NoiseParameters=[]  Unit=1  AffineConversion=off  FilteringAndDerivatives=zero  SimscapeFilterOrder=1  InputFilterTimeConstant=.001  UdotUserProvided=[]
  Simulink-PS Converter1 : nesl_utility/Simulink-PS Converter  PhysicalDomain=network_engine_domain  SubClassName=ps_input  LeftPortType=input  RightPortType=output  PseudoPeriodic=off  Frequencies=[]  NoiseDistribution=none  NoiseParameters=[]  Unit=1  AffineConversion=off  FilteringAndDerivatives=zero  SimscapeFilterOrder=1  InputFilterTimeConstant=.001  UdotUserProvided=[]
  Subsystem : Subsystem
  Sum : Sum  Inputs=|++
  To Workspace : ToWorkspace  VariableName=u_swing_ankle_data  SampleTime=-1
  To Workspace1 : ToWorkspace  VariableName=JointLimitTorqueSwingAnkle  SampleTime=-1
  To Workspace2 : ToWorkspace  VariableName=HardStopTorqueSwingAnkle  SampleTime=-1
  To Workspace5 : ToWorkspace  VariableName=TotalTorqueSwingAnkle  SampleTime=-1
  rad2deg : Gain  Gain=180/pi
  "rad2deg1 " : Gain  Gain=180/pi
  w : PMIOPort  Side=Right
  t : PMIOPort  Port=2  Side=Left
  q : PMIOPort  Port=3  Side=Right
  wires:
  PS-Simulink Converter1/1 -> "rad2deg1 "/1
  PS-Simulink Converter2/1 -> rad2deg/1
  rad2deg/1 -> Ankle_D_lookup/1, Scope7/1, Product/2, Ankle_S_lookup/1
  Ankle_S_lookup/1 -> Product/1
  "rad2deg1 "/1 -> Product1/1, Scope6/1
  Product1/1 -> Sum/1
  Product/1 -> Sum/2
  Sum/1 -> Gain/1
  Ankle_D_lookup/1 -> Product1/2
  Constant/1 -> Subsystem/1(u1)
  Constant1/1 -> Subsystem/2(u2)
  Constant2/1 -> Subsystem/3(u3)
  Constant3/1 -> Subsystem/4(u4)
  Constant4/1 -> Subsystem/5(u5)
  Subsystem/1(Out1) -> To Workspace/1, Simulink-PS Converter/1
  Constant5/1 -> Subsystem/6(u6)
  PS-Simulink Converter3/1 -> To Workspace2/1
  Gain/1 -> To Workspace1/1, Simulink-PS Converter1/1
  PS-Simulink Converter4/1 -> To Workspace5/1
  connections:
  w/RConn1 -- Hard_Stop_Ankle_L1/LConn1 -- PS-Simulink Converter1/LConn1
  Hard_Stop_Ankle_L1/RConn1 -- PS-Simulink Converter3/LConn1 -- PS Add/LConn2
  t/RConn1 -- PS-Simulink Converter4/LConn1 -- PS Add1/RConn1
  Simulink-PS Converter1/RConn1 -- PS Add1/LConn2
  q/RConn1 -- PS-Simulink Converter2/LConn1
  PS Add/RConn1 -- PS Add1/LConn1
  Simulink-PS Converter/RConn1 -- PS Add/LConn1

== system ss1_plant/Foot_L ==
  Ankle_L : sm_lib/Frames and Transforms/Rigid Transform  TranslationMethod=StandardAxis  TranslationStandardOffset=F_H  TranslationLengthUnit=m  TranslationStandardAxis=+Y  TranslationCartesianOffset=[0 0 0]  TranslationROffset=0  TranslationROffsetUnits=m  TranslationZOffset=0  TranslationZOffsetUnits=m  TranslationThetaOffset=0  TranslationThetaOffsetUnits=deg  RotationMethod=StandardAxis  RotationAngleUnits=deg  RotationStandardAxis=+Z  RotationAngle=-90  RotationArbitraryAxis=[0 0 1]  FollAlignAxisA=+Z  BaseAlignAxisA=+Z  FollAlignAxisB=+X  BaseAlignAxisB=+Y  RotationSequenceAxes=FollowerAxes  RotationSequence=XYX  RotationSequenceAngles=[0 0 0]  RotationSequenceAnglesUnits=deg  RotationMatrix=[1 0 0; 0 1 0; 0 0 1]
  Fcn : Fcn  Expr=180*atan(u(3)/(u(1)-u(2)))/pi
  Heel : sm_lib/Frames and Transforms/Rigid Transform  TranslationMethod=StandardAxis  TranslationStandardOffset=F_C  TranslationLengthUnit=m  TranslationStandardAxis=-X  TranslationCartesianOffset=[0 0 0]  TranslationROffset=0  TranslationROffsetUnits=m  TranslationZOffset=0  TranslationZOffsetUnits=m  TranslationThetaOffset=0  TranslationThetaOffsetUnits=deg  RotationMethod=AlignedAxes  RotationAngleUnits=deg  RotationStandardAxis=+Z  RotationAngle=0  RotationArbitraryAxis=[0 0 1]  FollAlignAxisA=+X  BaseAlignAxisA=+Z  FollAlignAxisB=+Y  BaseAlignAxisB=+X  RotationSequenceAxes=FollowerAxes  RotationSequence=XYX  RotationSequenceAngles=[0 0 0]  RotationSequenceAnglesUnits=deg  RotationMatrix=[1 0 0; 0 1 0; 0 0 1]
  Heel_GRF : Subsystem
  Mux : Mux  Inputs=3
  PS-Simulink Converter2 : nesl_utility/PS-Simulink Converter  PhysicalDomain=network_engine_domain  SubClassName=ps_output  LeftPortType=input  RightPortType=output  PseudoPeriodic=off  Frequencies=[]  Unit=1  AffineConversion=off
  PS-Simulink Converter3 : nesl_utility/PS-Simulink Converter  PhysicalDomain=network_engine_domain  SubClassName=ps_output  LeftPortType=input  RightPortType=output  PseudoPeriodic=off  Frequencies=[]  Unit=1  AffineConversion=off
  PS-Simulink Converter4 : nesl_utility/PS-Simulink Converter  PhysicalDomain=network_engine_domain  SubClassName=ps_output  LeftPortType=input  RightPortType=output  PseudoPeriodic=off  Frequencies=[]  Unit=1  AffineConversion=off
  Rigid  Transform : sm_lib/Frames and Transforms/Rigid Transform  TranslationMethod=StandardAxis  TranslationStandardOffset=T_R2  TranslationLengthUnit=m  TranslationStandardAxis=+Z  TranslationCartesianOffset=[0 0 0]  TranslationROffset=0  TranslationROffsetUnits=m  TranslationZOffset=0  TranslationZOffsetUnits=m  TranslationThetaOffset=0  TranslationThetaOffsetUnits=deg  RotationMethod=AlignedAxes  RotationAngleUnits=deg  RotationStandardAxis=+Z  RotationAngle=0  RotationArbitraryAxis=[0 0 1]  FollAlignAxisA=+X  BaseAlignAxisA=+Z  FollAlignAxisB=+Z  BaseAlignAxisB=+Y  RotationSequenceAxes=FollowerAxes  RotationSequence=XYX  RotationSequenceAngles=[0 0 0]  RotationSequenceAnglesUnits=deg  RotationMatrix=[1 0 0; 0 1 0; 0 0 1]
  Scope2 : Scope
  Solid : sm_lib/Body Elements/Solid  InertiaType=Custom  Mass=F_M  MassUnits=kg  CenterOfMass=[(F_L-F_C)/2, F_H/2, 0]  CenterOfMassUnits=m  MomentsOfInertia=[0.001 0.001 F_I]  MomentsOfInertiaUnits=kg*m^2  ProductsOfInertia=[0 0 0]  ProductsOfInertiaUnits=kg*m^2  BasedOnType=Density  Density=0  DensityUnits=kg/(m^3)  DoExposeReferenceFrame=on  SerializedFrames=<Frames/>  GraphicType=FromGeometry  MarkerShape=Sphere  MarkerSize=10  MarkerSizeUnits=m  GraphicVisPropType=SimpleVisualProperties  GraphicDiffuseColor=[0.0 0.4 1.0]  GraphicSpecularColor=[0.5 0.5 0.5 1.0]  GraphicAmbientColor=[0.15 0.15 0.15 1.0]  GraphicEmissiveColor=[0.0 0.0 0.0 1.0]  GraphicShininess=75  GraphicOpacity=1.0  GeometryShape=GeneralExtrusion  RectangleSize=[1 1]  RectangleSizeUnits=m  BrickDimensions=[1 1 1]  BrickDimensionUnits=m  CylinderRadius=1  CylinderRadiusUnits=m  CylinderLength=1  CylinderLengthUnits=m  SphereRadius=1  SphereRadiusUnits=m  EllipsoidRadii=[1 1 1]  EllipsoidRadiiUnits=m  ExtrusionCrossSection=F_cross_section  ExtrusionCrossSectionUnits=m  ExtrusionLength=F_W  ExtrusionLengthUnits=m  PolygonNumSides=3  PolygonOuterRadius=1  PolygonOuterRadiusUnits=m  ExtGeomFileType=STEP  ExtGeomFileUnits=m  RevolutionCrossSection=[1 1; 1 -1; 2 -1; 2 1]  RevolutionCrossSectionUnits=m  RevolutionExtent=Full  RevolutionAngle=180  RevolutionAngleUnits=deg
  Toe : sm_lib/Frames and Transforms/Rigid Transform  TranslationMethod=StandardAxis  TranslationStandardOffset=F_L-F_C  TranslationLengthUnit=m  TranslationStandardAxis=+X  TranslationCartesianOffset=[0 0 0]  TranslationROffset=0  TranslationROffsetUnits=m  TranslationZOffset=0  TranslationZOffsetUnits=m  TranslationThetaOffset=0  TranslationThetaOffsetUnits=deg  RotationMethod=AlignedAxes  RotationAngleUnits=deg  RotationStandardAxis=+Z  RotationAngle=0  RotationArbitraryAxis=[0 0 1]  FollAlignAxisA=+X  BaseAlignAxisA=+Z  FollAlignAxisB=+Y  BaseAlignAxisB=+X  RotationSequenceAxes=FollowerAxes  RotationSequence=XYX  RotationSequenceAngles=[0 0 0]  RotationSequenceAnglesUnits=deg  RotationMatrix=[1 0 0; 0 1 0; 0 0 1]
  Toe_GRF : Subsystem
  Transform  Sensor : sm_lib/Frames and Transforms/Transform Sensor  MeasurementFrame=World  SenseAngle=off  SenseAxis=off  SenseAngle1=off  SenseAngle2=off  SenseAngle3=off  SenseQ=off  SenseR=off  SenseOmegaX=off  SenseOmegaY=off  SenseOmegaZ=off  SenseOmega1=off  SenseOmega2=off  SenseOmega3=off  SenseQDot=off  SenseRDot=off  SenseAlphaX=off  SenseAlphaY=off  SenseAlphaZ=off  SenseAlpha1=off  SenseAlpha2=off  SenseAlpha3=off  SenseQDDot=off  SenseRDDot=off  SenseX=off  SenseY=on  SenseZ=off  SenseRad=off  SenseAzim=off  SenseDist=off  SenseInc=off  SenseXDot=off  SenseYDot=off  SenseZDot=off  SenseRadDot=off  SenseAzimDot=off  SenseDistDot=off  SenseIncDot=off  SenseXDDot=off  SenseYDDot=off  SenseZDDot=off  SenseRadDDot=off  SenseAzimDDot=off  SenseDistDDot=off  SenseIncDDot=off
  Transform  Sensor1 : sm_lib/Frames and Transforms/Transform Sensor  MeasurementFrame=World  SenseAngle=off  SenseAxis=off  SenseAngle1=off  SenseAngle2=off  SenseAngle3=off  SenseQ=off  SenseR=off  SenseOmegaX=off  SenseOmegaY=off  SenseOmegaZ=off  SenseOmega1=off  SenseOmega2=off  SenseOmega3=off  SenseQDot=off  SenseRDot=off  SenseAlphaX=off  SenseAlphaY=off  SenseAlphaZ=off  SenseAlpha1=off  SenseAlpha2=off  SenseAlpha3=off  SenseQDDot=off  SenseRDDot=off  SenseX=off  SenseY=on  SenseZ=on  SenseRad=off  SenseAzim=off  SenseDist=off  SenseInc=off  SenseXDot=off  SenseYDot=off  SenseZDot=off  SenseRadDot=off  SenseAzimDot=off  SenseDistDot=off  SenseIncDot=off  SenseXDDot=off  SenseYDDot=off  SenseZDDot=off  SenseRadDDot=off  SenseAzimDDot=off  SenseDistDDot=off  SenseIncDDot=off
  B : PMIOPort  Side=Right
  F : PMIOPort  Port=2  Side=Left
  F1 : PMIOPort  Port=3  Side=Left
  Stance_foot_orientation : Outport
  wires:
  PS-Simulink Converter3/1 -> Mux/1
  PS-Simulink Converter4/1 -> Mux/2
  PS-Simulink Converter2/1 -> Mux/3
  Mux/1 -> Fcn/1
  Fcn/1 -> Stance_foot_orientation/1, Scope2/1
  connections:
  B/RConn1 -- Rigid  Transform/RConn1
  Rigid  Transform/LConn1 -- Ankle_L/LConn1 -- Toe/LConn1 -- Heel/LConn1 -- Solid/RConn1 -- F1/RConn1
  Ankle_L/RConn1 -- F/RConn1
  Toe/RConn1 -- Transform  Sensor/RConn1 -- Toe_GRF/LConn1
  Heel/RConn1 -- Transform  Sensor1/RConn1 -- Heel_GRF/LConn1
  Transform  Sensor1/RConn3 -- PS-Simulink Converter2/LConn1
  Transform  Sensor1/RConn2 -- PS-Simulink Converter4/LConn1
  Transform  Sensor/RConn2 -- PS-Simulink Converter3/LConn1

== system ss1_plant/Foot_R ==
  Ankle_L : sm_lib/Frames and Transforms/Rigid Transform  TranslationMethod=StandardAxis  TranslationStandardOffset=F_H  TranslationLengthUnit=m  TranslationStandardAxis=+Y  TranslationCartesianOffset=[0 0 0]  TranslationROffset=0  TranslationROffsetUnits=m  TranslationZOffset=0  TranslationZOffsetUnits=m  TranslationThetaOffset=0  TranslationThetaOffsetUnits=deg  RotationMethod=StandardAxis  RotationAngleUnits=deg  RotationStandardAxis=+Z  RotationAngle=-90  RotationArbitraryAxis=[0 0 1]  FollAlignAxisA=+Z  BaseAlignAxisA=+Z  FollAlignAxisB=+X  BaseAlignAxisB=+Y  RotationSequenceAxes=FollowerAxes  RotationSequence=XYX  RotationSequenceAngles=[0 0 0]  RotationSequenceAnglesUnits=deg  RotationMatrix=[1 0 0; 0 1 0; 0 0 1]
  Heel : sm_lib/Frames and Transforms/Rigid Transform  TranslationMethod=StandardAxis  TranslationStandardOffset=F_C  TranslationLengthUnit=m  TranslationStandardAxis=-X  TranslationCartesianOffset=[0 0 0]  TranslationROffset=0  TranslationROffsetUnits=m  TranslationZOffset=0  TranslationZOffsetUnits=m  TranslationThetaOffset=0  TranslationThetaOffsetUnits=deg  RotationMethod=AlignedAxes  RotationAngleUnits=deg  RotationStandardAxis=+Z  RotationAngle=0  RotationArbitraryAxis=[0 0 1]  FollAlignAxisA=+X  BaseAlignAxisA=+Z  FollAlignAxisB=+Y  BaseAlignAxisB=+X  RotationSequenceAxes=FollowerAxes  RotationSequence=XYX  RotationSequenceAngles=[0 0 0]  RotationSequenceAnglesUnits=deg  RotationMatrix=[1 0 0; 0 1 0; 0 0 1]
  Rigid  Transform : sm_lib/Frames and Transforms/Rigid Transform  TranslationMethod=StandardAxis  TranslationStandardOffset=T_R2  TranslationLengthUnit=m  TranslationStandardAxis=+Z  TranslationCartesianOffset=[0 0 0]  TranslationROffset=0  TranslationROffsetUnits=m  TranslationZOffset=0  TranslationZOffsetUnits=m  TranslationThetaOffset=0  TranslationThetaOffsetUnits=deg  RotationMethod=AlignedAxes  RotationAngleUnits=deg  RotationStandardAxis=+Z  RotationAngle=0  RotationArbitraryAxis=[0 0 1]  FollAlignAxisA=+X  BaseAlignAxisA=+Z  FollAlignAxisB=+Z  BaseAlignAxisB=+Y  RotationSequenceAxes=FollowerAxes  RotationSequence=XYX  RotationSequenceAngles=[0 0 0]  RotationSequenceAnglesUnits=deg  RotationMatrix=[1 0 0; 0 1 0; 0 0 1]
  Solid : sm_lib/Body Elements/Solid  InertiaType=Custom  Mass=F_M  MassUnits=kg  CenterOfMass=[(F_L-F_C)/2, F_H/2, 0]  CenterOfMassUnits=m  MomentsOfInertia=[0.001 0.001 F_I]  MomentsOfInertiaUnits=kg*m^2  ProductsOfInertia=[0 0 0]  ProductsOfInertiaUnits=kg*m^2  BasedOnType=Density  Density=0  DensityUnits=kg/(m^3)  DoExposeReferenceFrame=on  SerializedFrames=<Frames/>  GraphicType=FromGeometry  MarkerShape=Sphere  MarkerSize=10  MarkerSizeUnits=m  GraphicVisPropType=SimpleVisualProperties  GraphicDiffuseColor=[0.0 0.4 1.0]  GraphicSpecularColor=[0.5 0.5 0.5 1.0]  GraphicAmbientColor=[0.15 0.15 0.15 1.0]  GraphicEmissiveColor=[0.0 0.0 0.0 1.0]  GraphicShininess=75  GraphicOpacity=1.0  GeometryShape=GeneralExtrusion  RectangleSize=[1 1]  RectangleSizeUnits=m  BrickDimensions=[1 1 1]  BrickDimensionUnits=m  CylinderRadius=1  CylinderRadiusUnits=m  CylinderLength=1  CylinderLengthUnits=m  SphereRadius=1  SphereRadiusUnits=m  EllipsoidRadii=[1 1 1]  EllipsoidRadiiUnits=m  ExtrusionCrossSection=F_cross_section  ExtrusionCrossSectionUnits=m  ExtrusionLength=F_W  ExtrusionLengthUnits=m  PolygonNumSides=3  PolygonOuterRadius=1  PolygonOuterRadiusUnits=m  ExtGeomFileType=STEP  ExtGeomFileUnits=m  RevolutionCrossSection=[1 1; 1 -1; 2 -1; 2 1]  RevolutionCrossSectionUnits=m  RevolutionExtent=Full  RevolutionAngle=180  RevolutionAngleUnits=deg
  Swing_foot_sensor : Subsystem
  To Workspace : ToWorkspace  VariableName=sl  SampleTime=-1
      settings: MaxDataPoints=1
  Toe : sm_lib/Frames and Transforms/Rigid Transform  TranslationMethod=StandardAxis  TranslationStandardOffset=F_L-F_C  TranslationLengthUnit=m  TranslationStandardAxis=+X  TranslationCartesianOffset=[0 0 0]  TranslationROffset=0  TranslationROffsetUnits=m  TranslationZOffset=0  TranslationZOffsetUnits=m  TranslationThetaOffset=0  TranslationThetaOffsetUnits=deg  RotationMethod=AlignedAxes  RotationAngleUnits=deg  RotationStandardAxis=+Z  RotationAngle=0  RotationArbitraryAxis=[0 0 1]  FollAlignAxisA=+X  BaseAlignAxisA=+Z  FollAlignAxisB=+Y  BaseAlignAxisB=+X  RotationSequenceAxes=FollowerAxes  RotationSequence=XYX  RotationSequenceAngles=[0 0 0]  RotationSequenceAnglesUnits=deg  RotationMatrix=[1 0 0; 0 1 0; 0 0 1]
  B : PMIOPort  Side=Right
  F : PMIOPort  Port=2  Side=Left
  swing_heel_z : Outport
  wires:
  Swing_foot_sensor/2(swing_heel_y) -> To Workspace/1
  Swing_foot_sensor/1(swing_heel_z) -> swing_heel_z/1
  connections:
  B/RConn1 -- Rigid  Transform/RConn1
  Swing_foot_sensor/LConn1 -- Swing_foot_sensor/LConn3 -- Swing_foot_sensor/LConn2 -- Solid/RConn1 -- Rigid  Transform/LConn1 -- Ankle_L/LConn1 -- Toe/LConn1 -- Heel/LConn1
  Ankle_L/RConn1 -- F/RConn1
